simulink model "BlocKDiagramReduced"  (R2024a)
settings: Solver=VariableStepAuto  StartTime=0.0  StopTime=10.0  RelTol=1e-3
values from neighbouring files (symbols this model uses):
  a1 = mw*Lw^2+If    (= 0.00856208)    [SystemVariablesForTransferFunction.m]
  a2 = (mf*Lf+mw*Lw)*g    (= 0.712409576)    [SystemVariablesForTransferFunction.m]
  Bf = 0.0036    [SystemVariablesForTransferFunction.m]
  Bw = 1.93*10^(-5)    (= 1.93e-05)    [SystemVariablesForTransferFunction.m]
  Iw = 699*10^(-6)    (= 0.000699)    [SystemVariablesForTransferFunction.m]
settings Model: Creator=gusta  LastModifiedBy=gusta

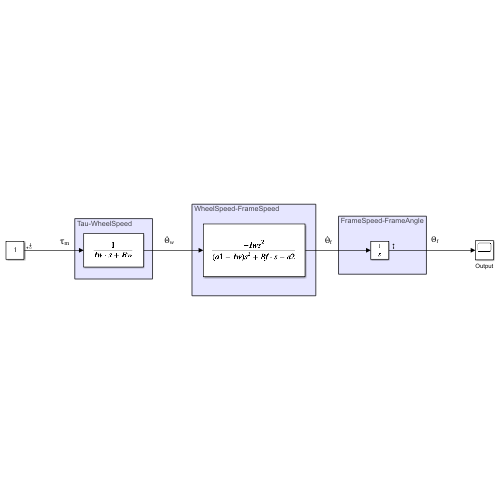
[thumbnail: Simulink's stored preview of the top-level diagram]
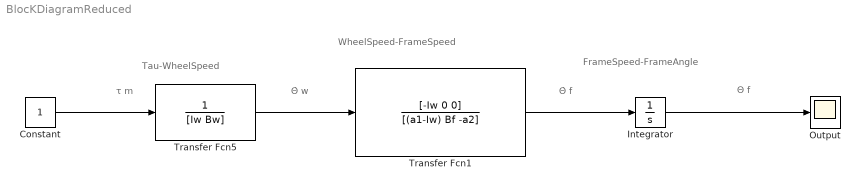
== system BlocKDiagramReduced ==
  note: FrameSpeed-FrameAngle
  note: Θ̇ f
  note: WheelSpeed-FrameSpeed
  note: Θ f
  note: τ m
  note: Θ̇ w
  note: Tau-WheelSpeed
  Constant : Constant
  Integrator : Integrator
  Output : Scope
  Transfer Fcn1 : TransferFcn  Numerator=[-Iw 0 0]  Denominator=[(a1-Iw) Bf -a2]
  Transfer Fcn5 : TransferFcn  Denominator=[Iw Bw]
  wires:
  Transfer Fcn1/1 -> Integrator/1
  Transfer Fcn5/1 -> Transfer Fcn1/1
  Integrator/1 -> Output/1
  Constant/1 -> Transfer Fcn5/1
